simulink subsystem "Day4_5_Scenario_1"  (R2024a)
settings: Solver=VariableStepAuto  StartTime=0.0  StopTime=10.0  RelTol=1e-3
libraries: CarMaker4SL x16, slpidlib x2
settings Model: Creator=junhyung.cha  LastModifiedBy=User

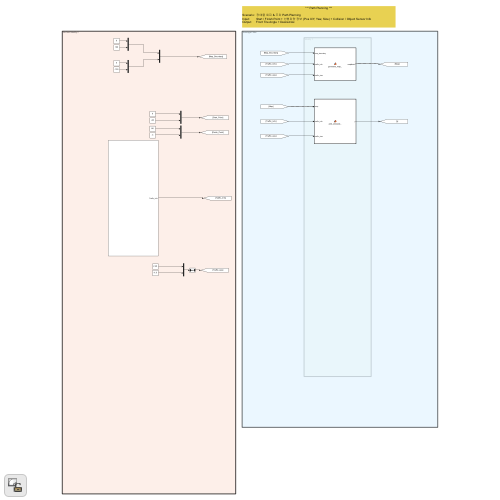
[thumbnail: Simulink's stored preview of the top-level diagram]
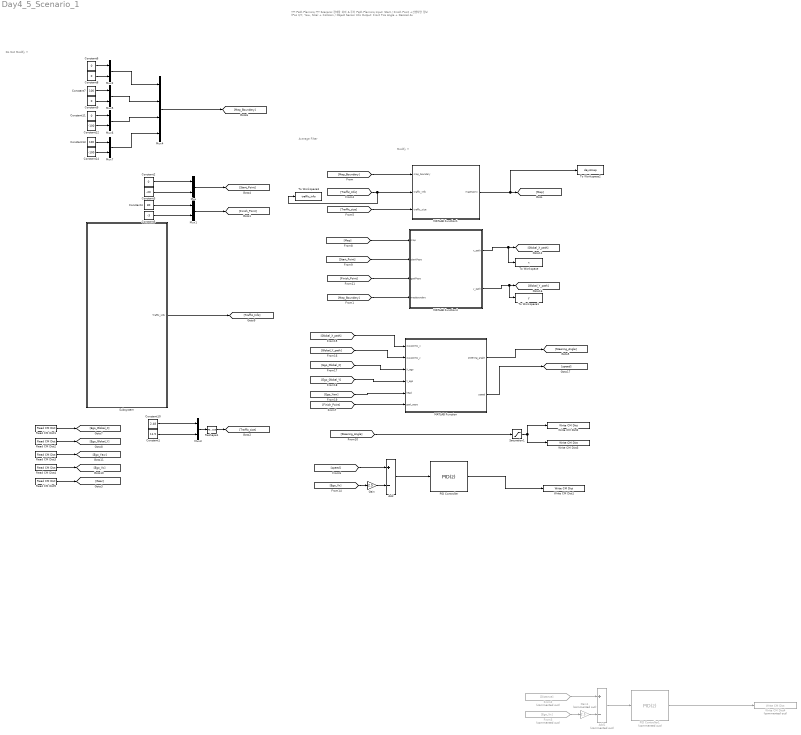
== system Day4_5_Scenario_1 ==
  note: Average Filter
  note: Do Not Modify !!
  note: Modify !!
  note: *** Path Planning ***
      |
      | Scenario: 장애물 회피 & 주차 Path Planning
      | Input: Start / Finish Point + 선행차량 정보 (Pos X/Y, Yaw, Size) + Collision / Object Sensor Info
      | Output: Front Tire Angle + Desired Ax
  Add : Sum  Inputs=+-
  Add1 : Sum  Commented=on  Inputs=+-
  Constant1 : Constant  Value=11.5
  Constant10 : Constant  Value=2.48
  Constant{2,6,8..9,11} (5 alike) : Constant  Value=0
  Constant12 : Constant  Value=-100
  Constant13 : Constant  Value=100
  Constant14 : Constant  Value=-100
  Constant3 : Constant  Value=-20
  Constant4 : Constant  Value=80
  Constant5 : Constant  Value=-3
  Constant7 : Constant  Value=100
  From2 : From  Commented=on  GotoTag=Distance
  From3 : From  Commented=on  GotoTag=Ego_Vx
  Gain : Gain  Gain=2.5
  Gain1 : Gain  Commented=on  Gain=2.5
  MATLAB Function : MATLAB Function  TreatAsAtomicUnit=on
  MATLAB Function1 : MATLAB Function  TreatAsAtomicUnit=on
  MATLAB Function4 : MATLAB Function  TreatAsAtomicUnit=on
  Mux{,1..3,5..7} (7 alike) : Mux  Inputs=2
  Mux4 : Mux
  PID Controller : slpidlib/PID Controller  Controller=PID  Form=Parallel  TimeDomain=Discrete-time  UseExternalTs=off  SampleTime=-1  IntegratorMethod=Forward Euler  FilterMethod=Forward Euler  ControllerParametersSource=internal  P=1  I=0  UseKiTs=off  D=0  UseExternalDerivativeSource=off  N=100  UseFilter=off  TunerSelectOption=Transfer Function Based (PID Tuner App)  InitialConditionSource=internal  InitialConditionForIntegrator=0  InitialConditionForFilter=0  DifferentiatorICPrevScaledInput=0  ExternalReset=none  TrackingMode=off  Kt=1  LimitOutput=off  SatLimitsSource=internal  UpperSaturationLimit=inf  LowerSaturationLimit=-inf  LinearizeAsGain=on  AntiWindupMode=none  Kb=1  LimitIntegrator=off  UpperIntegratorSaturationLimit=inf  LowerIntegratorSaturationLimit=-inf  POutMin=[]  POutMax=[]  IOutMin=[]  IOutMax=[]  DOutMin=[]  DOutMax=[]  NOutMin=[]  NOutMax=[]  SumOutMin=[]  SumOutMax=[]  SaturationOutMin=[]  SaturationOutMax=[]  PParamMin=[]  PParamMax=[]  IParamMin=[]  IParamMax=[]  DParamMin=[]  DParamMax=[]  NParamMin=[]  NParamMax=[]  KbParamMin=[]  KbParamMax=[]  KtParamMin=[]  KtParamMax=[]  KbOutMin=[]  KbOutMax=[]  KtOutMin=[]  KtOutMax=[]  IntegratorOutMin=[]  IntegratorOutMax=[]  FilterOutMin=[]  FilterOutMax=[]  SumI1OutMin=[]  SumI1OutMax=[]  SumI2OutMin=[]  SumI2OutMax=[]  SumI3OutMin=[]  SumI3OutMax=[]  SumI4OutMin=[]  SumI4OutMax=[]  SumDOutMin=[]  SumDOutMax=[]  DifferentiatorOutMin=[]  DifferentiatorOutMax=[]  FilterDiffOutCoefMin=[]  FilterDiffOutCoefMax=[]  ReciprocalOutMin=[]  ReciprocalOutMax=[]  SumDenOutMin=[]  SumDenOutMax=[]  SumNumOutMin=[]  SumNumOutMax=[]  DivideOutMin=[]  DivideOutMax=[]  UdiffTsProdOutMin=[]  UdiffTsProdOutMax=[]  NTsProdOutMin=[]  NTsProdOutMax=[]  UintegralTsProdOutMin=[]  UintegralTsProdOutMax=[]  UngainTsProdOutMin=[]  UngainTsProdOutMax=[]  ClampingZeroOutDataTypeStr=Inherit: Inherit via back propagation  ClampingZeroOutMin=[]  ClampingZeroOutMax=[]  FilterDenConstantOutDataTypeStr=Inherit: Inherit via back propagation  FilterDenConstantOutMin=[]  FilterDenConstantOutMax=[]  PCopyOutDataTypeStr=Inherit: Inherit via back propagation  PCopyOutMin=[]  PCopyOutMax=[]  NCopyOutDataTypeStr=Inherit: Inherit via back propagation  NCopyOutMin=[]  NCopyOutMax=[]  IntegratorContinuousStateAttributes=''  IntegratorStateMustResolveToSignalObject=off  IntegratorRTWStateStorageClass=Auto  FilterContinuousStateAttributes=''  FilterStateMustResolveToSignalObject=off  FilterRTWStateStorageClass=Auto  ParallelPVariant=InternalParameters  IdealPVariant=Disabled  IVariant=InternalParameters  DVariant=InternalParameters  IntegratorVariant=Discrete  SatVariant=Disabled  AWVariant=Passthrough  PCopyVariant=Disabled  TRVariant=Disabled  FdbkBlocksVariant=Forward  IdealPFdbkVariant=Disabled  SatFdbkVariant=Disabled  DerivativeFilterVariant=Differentiator  NVariant=Passthrough  NCopyVariant=Disabled_SignalSpec  FilterICVariant=InternalICsDifferentiator  IntegratorICVariant=InternalICs  ExternalResetVariant=Disabled  TRSumVariant=Passthrough  SumFdbkVariant=Disabled  SumVariant=Sum_PID  TsampFilterVariant=InternalTs  TsampNgainVariant=Passthrough  TsampIntegralVariant=Disabled_SignalSpec  ExternalSaturationOutDataTypeStr=Inherit: Same as second input  DerivativeSourceVariant=ErrorSignal
  PID Controller1 : slpidlib/PID Controller  Commented=on  Controller=PID  Form=Parallel  TimeDomain=Discrete-time  UseExternalTs=off  SampleTime=-1  IntegratorMethod=Forward Euler  FilterMethod=Forward Euler  ControllerParametersSource=internal  P=5  I=0  UseKiTs=off  D=0  UseExternalDerivativeSource=off  N=100  UseFilter=off  TunerSelectOption=Transfer Function Based (PID Tuner App)  InitialConditionSource=internal  InitialConditionForIntegrator=0  InitialConditionForFilter=0  DifferentiatorICPrevScaledInput=0  ExternalReset=none  TrackingMode=off  Kt=1  LimitOutput=off  SatLimitsSource=internal  UpperSaturationLimit=inf  LowerSaturationLimit=-inf  LinearizeAsGain=on  AntiWindupMode=none  Kb=1  LimitIntegrator=off  UpperIntegratorSaturationLimit=inf  LowerIntegratorSaturationLimit=-inf  POutMin=[]  POutMax=[]  IOutMin=[]  IOutMax=[]  DOutMin=[]  DOutMax=[]  NOutMin=[]  NOutMax=[]  SumOutMin=[]  SumOutMax=[]  SaturationOutMin=[]  SaturationOutMax=[]  PParamMin=[]  PParamMax=[]  IParamMin=[]  IParamMax=[]  DParamMin=[]  DParamMax=[]  NParamMin=[]  NParamMax=[]  KbParamMin=[]  KbParamMax=[]  KtParamMin=[]  KtParamMax=[]  KbOutMin=[]  KbOutMax=[]  KtOutMin=[]  KtOutMax=[]  IntegratorOutMin=[]  IntegratorOutMax=[]  FilterOutMin=[]  FilterOutMax=[]  SumI1OutMin=[]  SumI1OutMax=[]  SumI2OutMin=[]  SumI2OutMax=[]  SumI3OutMin=[]  SumI3OutMax=[]  SumI4OutMin=[]  SumI4OutMax=[]  SumDOutMin=[]  SumDOutMax=[]  DifferentiatorOutMin=[]  DifferentiatorOutMax=[]  FilterDiffOutCoefMin=[]  FilterDiffOutCoefMax=[]  ReciprocalOutMin=[]  ReciprocalOutMax=[]  SumDenOutMin=[]  SumDenOutMax=[]  SumNumOutMin=[]  SumNumOutMax=[]  DivideOutMin=[]  DivideOutMax=[]  UdiffTsProdOutMin=[]  UdiffTsProdOutMax=[]  NTsProdOutMin=[]  NTsProdOutMax=[]  UintegralTsProdOutMin=[]  UintegralTsProdOutMax=[]  UngainTsProdOutMin=[]  UngainTsProdOutMax=[]  ClampingZeroOutDataTypeStr=Inherit: Inherit via back propagation  ClampingZeroOutMin=[]  ClampingZeroOutMax=[]  FilterDenConstantOutDataTypeStr=Inherit: Inherit via back propagation  FilterDenConstantOutMin=[]  FilterDenConstantOutMax=[]  PCopyOutDataTypeStr=Inherit: Inherit via back propagation  PCopyOutMin=[]  PCopyOutMax=[]  NCopyOutDataTypeStr=Inherit: Inherit via back propagation  NCopyOutMin=[]  NCopyOutMax=[]  IntegratorContinuousStateAttributes=''  IntegratorStateMustResolveToSignalObject=off  IntegratorRTWStateStorageClass=Auto  FilterContinuousStateAttributes=''  FilterStateMustResolveToSignalObject=off  FilterRTWStateStorageClass=Auto  ParallelPVariant=InternalParameters  IdealPVariant=Disabled  IVariant=InternalParameters  DVariant=InternalParameters  IntegratorVariant=Discrete  SatVariant=Disabled  AWVariant=Passthrough  PCopyVariant=Disabled  TRVariant=Disabled  FdbkBlocksVariant=Forward  IdealPFdbkVariant=Disabled  SatFdbkVariant=Disabled  DerivativeFilterVariant=Differentiator  NVariant=Passthrough  NCopyVariant=Disabled_SignalSpec  FilterICVariant=InternalICsDifferentiator  IntegratorICVariant=InternalICs  ExternalResetVariant=Disabled  TRSumVariant=Passthrough  SumFdbkVariant=Disabled  SumVariant=Sum_PID  TsampFilterVariant=InternalTs  TsampNgainVariant=Passthrough  TsampIntegralVariant=Disabled_SignalSpec  ExternalSaturationOutDataTypeStr=Inherit: Same as second input  DerivativeSourceVariant=ErrorSignal
  Read CM Dict1 : CarMaker4SL/Read CM Dict  xname=Car.Fr1.tx  xsync=off  xstime=Inherited
  Read CM Dict2 : CarMaker4SL/Read CM Dict  xname=Car.Fr1.ty  xsync=off  xstime=Inherited
  Read CM Dict3 : CarMaker4SL/Read CM Dict  xname=Car.Fr1.rz  xsync=off  xstime=Inherited
  Read CM Dict4 : CarMaker4SL/Read CM Dict  xname=Car.v  xsync=off  xstime=Inherited
  Read CM Dict5 : CarMaker4SL/Read CM Dict  xname=DM.SelectorCtrl  xsync=off  xstime=Inherited
  Reshape1 : Reshape  OutputDimensionality=Row vector (2-D)  OutputDimensions=[2,2]
  Saturation1 : Saturate  UpperLimit=pi/6  LowerLimit=-pi/6
  Subsystem : Subsystem
  To Workspace : ToWorkspace  VariableName=x  SaveFormat=Timeseries  SampleTime=-1
  To Workspace1 : ToWorkspace  VariableName=y  SaveFormat=Timeseries  SampleTime=-1
  To Workspace2 : ToWorkspace  VariableName=day4map  SaveFormat=Timeseries  SampleTime=-1
  To Workspace3 : ToWorkspace  VariableName=traffic_info  SaveFormat=Timeseries  SampleTime=-1
  Write CM Dict1 : CarMaker4SL/Write CM Dict  xname=AccelCtrl.DesiredAx  xsync=off
  Write CM Dict2 : CarMaker4SL/Write CM Dict  xname=Car.CFL.rz_ext  xsync=off
  Write CM Dict3 : CarMaker4SL/Write CM Dict  xname=Car.CFR.rz_ext  xsync=off
  Write CM Dict4 : CarMaker4SL/Write CM Dict  Commented=on  xname=AccelCtrl.DesiredAx  xsync=off
  wires:
  Mux/1 -> [Start_Point]
  Constant2/1 -> Mux/1
  Constant3/1 -> Mux/2
  Constant5/1 -> Mux1/2
  Mux1/1 -> [Finish_Point]
  Constant4/1 -> Mux1/1
  Constant6/1 -> Mux2/1
  Constant8/1 -> Mux2/2
  Constant9/1 -> Mux5/2
  [Map_Boundary] -> MATLAB Function1/1(map_boundary)
  Subsystem/1(Traffic_Info) -> [Traffic_Info]
  Mux3/1 -> Reshape1/1
  Constant10/1 -> Mux3/1
  Constant1/1 -> Mux3/2
  Mux2/1 -> Mux4/1
  Mux5/1 -> Mux4/2
  Mux4/1 -> [Map_Boundary]
  Constant7/1 -> Mux5/1
  [Traffic_Info] -> MATLAB Function1/2(traffic_info), To Workspace3/1
  Reshape1/1 -> [Traffic_size]
  MATLAB Function1/1(mapMatrix) -> [Map], To Workspace2/1
  Read CM Dict2/1 -> [Ego_Global_Y]
  Read CM Dict1/1 -> [Ego_Global_X]
  Read CM Dict4/1 -> [Ego_Vx]
  Read CM Dict3/1 -> [Ego_Yaw]
  Saturation1/1 -> Write CM Dict3/1, Write CM Dict2/1
  [Steering_Angle] -> Saturation1/1
  Add/1 -> PID Controller/1
  Constant11/1 -> Mux6/1
  Constant12/1 -> Mux6/2
  Constant13/1 -> Mux7/1
  Constant14/1 -> Mux7/2
  Mux6/1 -> Mux4/3
  Mux7/1 -> Mux4/4
  [Ego_Yaw] -> MATLAB Function/5(head)
  [Global_X_path] -> MATLAB Function/1(waypoints_x)
  [Global_Y_path] -> MATLAB Function/2(waypoints_y)
  [Ego_Global_X] -> MATLAB Function/3(X_ego)
  [Ego_Global_Y] -> MATLAB Function/4(Y_ego)
  [Map] -> MATLAB Function4/1(map)
  [Start_Point] -> MATLAB Function4/2(startPose)
  [Finish_Point] -> MATLAB Function4/3(goalPose)
  MATLAB Function4/2(y_path) -> [Global_Y_path], To Workspace1/1
  [Map_Boundary] -> MATLAB Function4/4(mapboundary)
  MATLAB Function4/1(x_path) -> [Global_X_path], To Workspace/1
  MATLAB Function/1(steering_angle) -> [Steering_Angle]
  Gain1/1 -> Add1/2
  Add1/1 -> PID Controller1/1
  From2/1 -> Add1/1
  From3/1 -> Gain1/1
  PID Controller1/1 -> Write CM Dict4/1
  [Ego_Vx] -> Gain/1
  Gain/1 -> Add/2
  [Finish_Point] -> MATLAB Function/6(goal_pose)
  MATLAB Function/2(speed) -> [speed]
  [speed] -> Add/1
  Read CM Dict5/1 -> [Gear]
  PID Controller/1 -> Write CM Dict1/1
  [Traffic_size] -> MATLAB Function1/3(traffic_size)

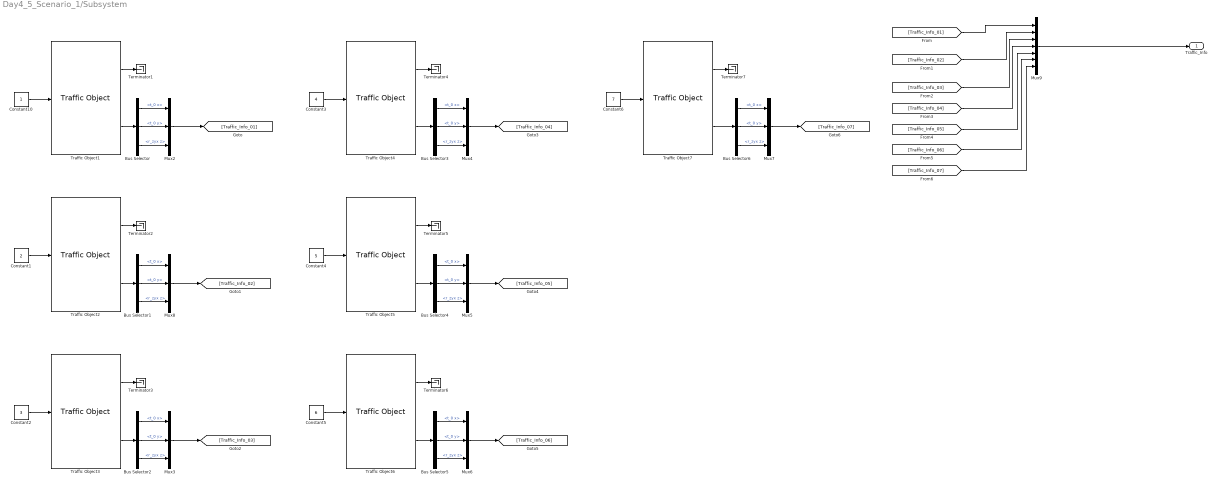
== system Day4_5_Scenario_1/Subsystem ==
  Bus Selector{,1..6} (7 alike) : BusSelector  OutputSignals=t_0 x,t_0 y,r_zyx z
  Constant1 : Constant  Value=2
  Constant10 : Constant
  Constant2 : Constant  Value=3
  Constant3 : Constant  Value=4
  Constant4 : Constant  Value=5
  Constant5 : Constant  Value=6
  Constant6 : Constant  Value=7
  Mux{2..8} (7 alike) : Mux  Inputs=3
  Mux9 : Mux  Inputs=7
  Terminator{1..7} (7 alike) : Terminator
  Traffic Object1 : CarMaker4SL/Traffic Object  xname=T01  ximode=Traffic Id  xstime=Inherited
      settings: SourceProductName=CarMaker4SL
  Traffic Object2 : CarMaker4SL/Traffic Object  xname=T02  ximode=Traffic Id  xstime=Inherited
      settings: SourceProductName=CarMaker4SL
  Traffic Object3 : CarMaker4SL/Traffic Object  xname=T03  ximode=Traffic Id  xstime=Inherited
      settings: SourceProductName=CarMaker4SL
  Traffic Object4 : CarMaker4SL/Traffic Object  xname=T04  ximode=Traffic Id  xstime=Inherited
      settings: SourceProductName=CarMaker4SL
  Traffic Object5 : CarMaker4SL/Traffic Object  xname=T05  ximode=Traffic Id  xstime=Inherited
      settings: SourceProductName=CarMaker4SL
  Traffic Object6 : CarMaker4SL/Traffic Object  xname=T06  ximode=Traffic Id  xstime=Inherited
      settings: SourceProductName=CarMaker4SL
  Traffic Object7 : CarMaker4SL/Traffic Object  xname=T07  ximode=Traffic Id  xstime=Inherited
      settings: SourceProductName=CarMaker4SL
  Traffic_Info : Outport
  wires:
  [Traffic_Info_07] -> Mux9/7
  [Traffic_Info_06] -> Mux9/6
  [Traffic_Info_05] -> Mux9/5
  [Traffic_Info_04] -> Mux9/4
  [Traffic_Info_03] -> Mux9/3
  Mux9/1 -> Traffic_Info/1
  [Traffic_Info_02] -> Mux9/2
  [Traffic_Info_01] -> Mux9/1
  Mux2/1 -> [Traffic_Info_01]
  Traffic Object7/2 -> Bus Selector6/1
  Bus Selector6/3 -> Mux7/3  "<r_zyx z>"
  Bus Selector6/1 -> Mux7/1  "<t_0 x>"
  Mux7/1 -> [Traffic_Info_07]
  Bus Selector6/2 -> Mux7/2  "<t_0 y>"
  Traffic Object6/2 -> Bus Selector5/1
  Bus Selector5/3 -> Mux6/3  "<r_zyx z>"
  Bus Selector5/1 -> Mux6/1  "<t_0 x>"
  Mux6/1 -> [Traffic_Info_06]
  Bus Selector5/2 -> Mux6/2  "<t_0 y>"
  Traffic Object5/2 -> Bus Selector4/1
  Bus Selector4/3 -> Mux5/3  "<r_zyx z>"
  Bus Selector4/1 -> Mux5/1  "<t_0 x>"
  Mux5/1 -> [Traffic_Info_05]
  Bus Selector4/2 -> Mux5/2  "<t_0 y>"
  Traffic Object4/2 -> Bus Selector3/1
  Bus Selector3/3 -> Mux4/3  "<r_zyx z>"
  Bus Selector3/1 -> Mux4/1  "<t_0 x>"
  Mux4/1 -> [Traffic_Info_04]
  Bus Selector3/2 -> Mux4/2  "<t_0 y>"
  Traffic Object3/2 -> Bus Selector2/1
  Bus Selector2/3 -> Mux3/3  "<r_zyx z>"
  Bus Selector2/1 -> Mux3/1  "<t_0 x>"
  Mux3/1 -> [Traffic_Info_03]
  Bus Selector2/2 -> Mux3/2  "<t_0 y>"
  Traffic Object2/2 -> Bus Selector1/1
  Bus Selector1/3 -> Mux8/3  "<r_zyx z>"
  Bus Selector1/1 -> Mux8/1  "<t_0 x>"
  Mux8/1 -> [Traffic_Info_02]
  Bus Selector1/2 -> Mux8/2  "<t_0 y>"
  Bus Selector/3 -> Mux2/3  "<r_zyx z>"
  Bus Selector/2 -> Mux2/2  "<t_0 y>"
  Bus Selector/1 -> Mux2/1  "<t_0 x>"
  Traffic Object1/2 -> Bus Selector/1
  Traffic Object7/1 -> Terminator7/1
  Constant6/1 -> Traffic Object7/1
  Constant5/1 -> Traffic Object6/1
  Traffic Object6/1 -> Terminator6/1
  Traffic Object5/1 -> Terminator5/1
  Constant4/1 -> Traffic Object5/1
  Constant3/1 -> Traffic Object4/1
  Traffic Object4/1 -> Terminator4/1
  Traffic Object3/1 -> Terminator3/1
  Constant2/1 -> Traffic Object3/1
  Constant1/1 -> Traffic Object2/1
  Traffic Object2/1 -> Terminator2/1
  Traffic Object1/1 -> Terminator1/1
  Constant10/1 -> Traffic Object1/1

== matlab function Day4_5_Scenario_1/MATLAB Function ==
  settings: updateMethod=DISCRETE  sampleTime=1
  data: waypoints_x input; waypoints_y input; X_ego input; Y_ego input; head input; steering_angle output; goal_pose input; speed output
function [steering_angle, speed] = ...
    global_to_local_waypoints(waypoints_x, waypoints_y, ...
                              X_ego, Y_ego, head, goal_pose)
%#codegen
% 글로벌 웨이포인트 → 로컬 좌표 변환 + 조향각 계산 (Pure Pursuit)
% 후방 포인트는 무시하며, 초기에는 아무 유효 포인트 없을 수 있음

    %% 파라미터
    L = 4.0;               % 휠베이스
    epsilon = 1e-3;        % 안정화용
    lookahead_dist = 1.0;  % 추적 기준 거리
    stop_threshold = 2.8;  % 완전 정지 거리
    heading_align_threshold = 15.0;  % 헤딩 조정 시작 거리

    %% 초기값 설정 (모든 실행 경로 보장)
    local_point = [0 0];
    dist = 0;
    idx_closest = 1;
    steering_angle = 0;
    goal_dist = norm([X_ego - goal_pose(1), Y_ego - goal_pose(2)]);
    
    %% 정지 조건
    if goal_dist < stop_threshold
        speed = 0;
        steering_angle = 0;
        return;
    end

    %% 헤딩 정렬 조건 적용
    if goal_dist < heading_align_threshold
        heading_error = wrapToPi(pi/2 - head);  % 90도 방향으로 정렬
        steering_angle = atan2(2 * L * sin(heading_error), goal_dist + epsilon);
        speed = 0;
        % 이 부분에서 
        return;
    end

    %% 1) NaN 제거
    valid_idx = ~isnan(waypoints_x) & ~isnan(waypoints_y);
    x_wp = waypoints_x(valid_idx);
    y_wp = waypoints_y(valid_idx);
    N = numel(x_wp);

    if N == 0
        speed = 0;
        return;
    end

    %% 2) 차량 기준 상대 위치 계산
    dx_all = x_wp(:)' - X_ego;
    dy_all = y_wp(:)' - Y_ego;

    %% 3) 차량 전방 필터
    forward_vec = [cos(head); sin(head)];
    rel_pos = [dx_all; dy_all];
    dot_products = forward_vec' * rel_pos;
    is_in_front = dot_products > 0;

    %% 4) 전방 포인트가 없다면: 정지 상태 유지
    if ~any(is_in_front)
        speed = 0;
        return;
    end

    %% 5) 가장 가까운 전방 인덱스 찾기
    d2_all = dx_all.^2 + dy_all.^2;
    d2_all(~is_in_front) = Inf;
    [~, idx_closest] = min(d2_all);

    %% 6) 전체 로컬 좌표 변환
    c = cos(-head); s = sin(-head);
    R = [c, -s; s, c];
    rel_global = [x_wp - X_ego, y_wp - Y_ego]';
    local_wp = R * rel_global;       % 2×N
    Local_Waypoints = local_wp';     % Nx2
    local_point = Local_Waypoints(idx_closest, :);
    dist = sqrt(d2_all(idx_closest));

    %% 7) 추적 포인트 찾기 (lookahead 거리 기준)
    target_idx = idx_closest;
    for i = idx_closest+1:N
        d = norm(Local_Waypoints(i,:) - Local_Waypoints(idx_closest,:));
        if d > lookahead_dist
            target_idx = i;
            break;
        end
    end

    %% 8) 조향각 계산 (Pure Pursuit)
    x_t = Local_Waypoints(target_idx, 1);
    y_t = Local_Waypoints(target_idx, 2);
    L_d = sqrt(x_t^2 + y_t^2 + epsilon);
    alpha = atan2(y_t, x_t);
    steering_angle = atan2(2 * L * sin(alpha), L_d);

    %% 9) 속도 설정
    speed = 10;
end

%% ===== 각도 wrap =====
function angle = wrapToPi(theta)
    angle = mod(theta + pi, 2*pi) - pi;
end

== matlab function Day4_5_Scenario_1/MATLAB Function4 ==
  settings: updateMethod=DISCRETE  sampleTime=1
  data: map input; x_path output; startPose input; goalPose input; y_path output; mapboundary input
function [x_path, y_path] = rrt_star_planner(map, startPose, goalPose, mapboundary)
    %% ===== Persistent 저장 =====
    persistent path_initialized x_path_cached y_path_cached nPath_cached
    maxPathLength = 500;
    resolution = 1;

    if isempty(path_initialized)
        path_initialized = false;
        x_path_cached = zeros(maxPathLength, 1);
        y_path_cached = zeros(maxPathLength, 1);
        nPath_cached = 1;
    end

    if path_initialized
        x_path = x_path_cached(1:nPath_cached);
        y_path = y_path_cached(1:nPath_cached);
        return;
    end

    %% 설정
    visualize      = false;
    maxIter        = 5000;
    stepSize       = 2;
    goalSampleRate = 0.1;
    successDistTh  = 5;
    collisionRes   = 0.5;
    searchRadius   = 10;
    safetyDist     = 13;

    %% 바운더리 기반 인덱스 변환용 파라미터
    x_values = mapboundary(1:2:end)
    y_values = mapboundary(2:2:end);
    x_min = min(x_values);
    y_max = max(y_values);

    %% 실좌표 → 인덱스 변환
    toGrid = @(x, y) [(x - x_min)/resolution + 1, (y_max - y)/resolution + 1];

    start_grid = toGrid(startPose(1), startPose(2));
    goal_grid  = toGrid(goalPose(1), goalPose(2));

    %% 트리 초기화 (모든 노드는 인덱스 좌표로 유지)
    nodes = struct('x', start_grid(1), 'y', start_grid(2), ...
                   'parent', 0, 'cost', 0);

    %% 경로 및 출력 초기화
    path   = struct('x', {}, 'y', {}, 'parent', {}, 'cost', {});
    x_path = zeros(maxPathLength, 1);
    y_path = zeros(maxPathLength, 1);

    %% RRT* 메인 루프 (모든 연산 인덱스 기반)
    for iter = 1:maxIter
        if rand < goalSampleRate
            xr = goal_grid;
        else
            xr = [randi([1, size(map,2)]), randi([1, size(map,1)])];
        end

        [nearestIdx, nearXY] = findNearest(nodes, xr);
        theta = atan2(xr(2)-nearXY(2), xr(1)-nearXY(1));
        newXY = nearXY + stepSize * [cos(theta), sin(theta)];

        if isCollision(newXY, map) || ...
           isPathCollision(nearXY, newXY, map, collisionRes) || ...
           isNearObstacle(newXY, map, safetyDist)
            continue;
        end

        nearIdxs = findNearNodes(nodes, newXY, searchRadius);
        minCost   = nodes(nearestIdx).cost + norm(newXY - nearXY);
        minParent = nearestIdx;

        for idx = 1:numel(nearIdxs)
            iNode = nearIdxs(idx);
            pxy   = [nodes(iNode).x, nodes(iNode).y];
            if ~isPathCollision(pxy, newXY, map, collisionRes)
                c = nodes(iNode).cost + norm(newXY - pxy);
                if c < minCost
                    minCost   = c;
                    minParent = iNode;
                end
            end
        end

        newNode = struct('x', newXY(1), 'y', newXY(2), ...
                         'parent', minParent, 'cost', minCost);
        nodes(end+1) = newNode;
        newIdx       = numel(nodes);

        for idx = 1:numel(nearIdxs)
            iNode = nearIdxs(idx);
            pxy   = [nodes(iNode).x, nodes(iNode).y];
            c     = newNode.cost + norm([newNode.x, newNode.y] - pxy);
            if c < nodes(iNode).cost && ...
               ~isPathCollision([newNode.x,newNode.y], pxy, map, collisionRes)
                nodes(iNode).parent = newIdx;
                nodes(iNode).cost   = c;
            end
        end

        if visualize
            plot([nodes(newNode.parent).x, newNode.x], ...
                 [nodes(newNode.parent).y, newNode.y], '-r');
            hold on;
        end

        if norm(newXY - goal_grid) < successDistTh
            if visualize, disp('[-] GOAL REACHED'); end
            path = backtrace(nodes, newIdx);
            break;
        end
    end

    %% 결과 경로 반환 (인덱스 → 실좌표로 역변환)
    nPath = min(numel(path), maxPathLength);
    x_path_cached = zeros(maxPathLength, 1);
    y_path_cached = zeros(maxPathLength, 1);
    for k = 1:nPath
        x_path_cached(k) = (path(k).x - 1) * resolution + x_min;
        y_path_cached(k) = y_max - (path(k).y - 1) * resolution;
    end

    nPath_cached = nPath;
    path_initialized = true;

    %% === Lightweight Smoothing for Simulink Compatibility ===
    smooth_window = 15;  % 홀수 추천
    if nPath >= smooth_window
        x = x_path_cached(1:nPath);
        y = y_path_cached(1:nPath);

        x_smooth = movmean(x, smooth_window);
        y_smooth = movmean(y, smooth_window);

        % 재샘플링 (고정된 개수로)
        smoothN = 100;
        idx_original = linspace(1, numel(x_smooth), smoothN);
        x_path = interp1(1:numel(x_smooth), x_smooth, idx_original, 'linear')';
        y_path = interp1(1:numel(y_smooth), y_smooth, idx_original, 'linear')';
    else
        x_path = x_path_cached(1:nPath);
        y_path = y_path_cached(1:nPath);
    end


end

%% ======= 서브 함수들 =======

function [idx, xy] = findNearest(nodes, sampleXY)
    d = arrayfun(@(n) hypot(n.x - sampleXY(1), n.y - sampleXY(2)), nodes);
    [~, idx] = min(d);
    xy = [nodes(idx).x, nodes(idx).y];
end

function nearIdxs = findNearNodes(nodes, pos, radius)
    maxNodes = 1000;
    nearIdxs = zeros(1, maxNodes);
    count = 0;
    for i = 1:numel(nodes)
        if hypot(nodes(i).x - pos(1), nodes(i).y - pos(2)) <= radius
            count = count + 1;
            nearIdxs(count) = i;
        end
    end
    nearIdxs = nearIdxs(1:count);
end

function flag = isCollision(pt, map)
    x = round(pt(1)); y = round(pt(2));
    flag = x < 1 || x > size(map,2) || y < 1 || y > size(map,1) || map(y,x) == 1;
end

function flag = isPathCollision(p1, p2, map, step)
    dist = norm(p2 - p1);
    N = max(1, ceil(dist / step));
    flag = false;
    for i = 0:N
        pt = p1 + (p2 - p1) * (i / N);
        if isCollision(pt, map)
            flag = true; return;
        end
    end
end

function flag = isNearObstacle(pt, map, safeDist)
    x0 = round(pt(1)); y0 = round(pt(2));
    r  = ceil(safeDist);
    [X, Y] = meshgrid((x0 - r):(x0 + r), (y0 - r):(y0 + r));
    D2 = (X - pt(1)).^2 + (Y - pt(2)).^2;
    mask = D2 <= safeDist^2;
    X = X(mask); Y = Y(mask);
    valid = X >= 1 & X <= size(map,2) & Y >= 1 & Y <= size(map,1);
    flag  = any(map(sub2ind(size(map), Y(valid), X(valid))) == 1);
end

function path = backtrace(nodes, idx)
    maxPathLen = 500;
    dummyNode = struct('x', 0, 'y', 0, 'parent', 0, 'cost', 0);
    path = repmat(dummyNode, maxPathLen, 1);
    count = 0;
    while idx ~= 0 && count < maxPathLen
        count = count + 1;
        path(count) = nodes(idx);
        idx = nodes(idx).parent;
    end
    path = path(count:-1:1);
end

== matlab function Day4_5_Scenario_1/MATLAB Function1 ==
  settings: updateMethod=DISCRETE  sampleTime=1
  data: map_boundary input; mapMatrix output size=[1000, 1000]; traffic_info input; traffic_size input
%% ======== generate_map_ ======== Ver 2025-05-17 10:40 (persistent 적용)
function mapMatrix = generate_map_(map_boundary, traffic_info, traffic_size)
    %— persistent로 첫 실행 여부와 결과 저장
    % persistent stopped
    % 
    % if isempty(stopped)
    %     stopped = false;
    % end
    % if stopped
    %     return;
    % end
    traffic_info_mat = reshape(traffic_info, 3, []).';
    resolution = 1;
    x_values = map_boundary(1:2:end);
    y_values = map_boundary(2:2:end);
    N = size(traffic_info_mat,1);
    w = traffic_size(1);
    h = traffic_size(2);
    x_min = min(x_values);  x_max = max(x_values);
    y_min = min(y_values);  y_max = max(y_values);
    x_size = ceil((x_max-x_min)/resolution);
    y_size = ceil((y_max-y_min)/resolution);
    
    
    mapMatrix = zeros(y_size, x_size); %출력코드
    
    for i = 1:N
        x_c = traffic_info_mat(i, 1);
        y_c = traffic_info_mat(i, 2);
        yaw = traffic_info_mat(i, 3);
        
        dx = w/2;  dy = h/2;
        local = [-dx,-dy; dx,-dy; dx,dy; -dx,dy];
        R = [cos(yaw), -sin(yaw); sin(yaw), cos(yaw)];
        rotated = (R*local')';
        forward_vec = [cos(yaw), sin(yaw)];
        side_vec    = [-sin(yaw), cos(yaw)];
        center = [x_c, y_c] + (w/2)*forward_vec - (h/2)*side_vec;
        corners = rotated + center;
        x_idx = (corners(:,1)-x_min)/resolution + 1;
        y_idx = (y_max-corners(:,2))/resolution + 1;
        mask = poly2mask(x_idx, y_idx, y_size, x_size);
        mapMatrix(mask) = 1;
    end
    %mapMatrix_stored = mapMatrix;
    % stopped = true;
end
